simulink model "Drone_Sim"  (R2019b)
settings: Solver=ode15s  StartTime=0.0  StopTime=20  FixedStep=0.1
libraries: simulink x7
settings Model: Creator=harry  LastModifiedBy=cj
settings DataIOCC: ReturnWorkspaceOutputs=off
settings DebuggingCC: ArithmeticOperatorsInVariantConditions=warning
settings SFSimCC: CustomCodeUndefinedFunction=UseInterfaceOnly

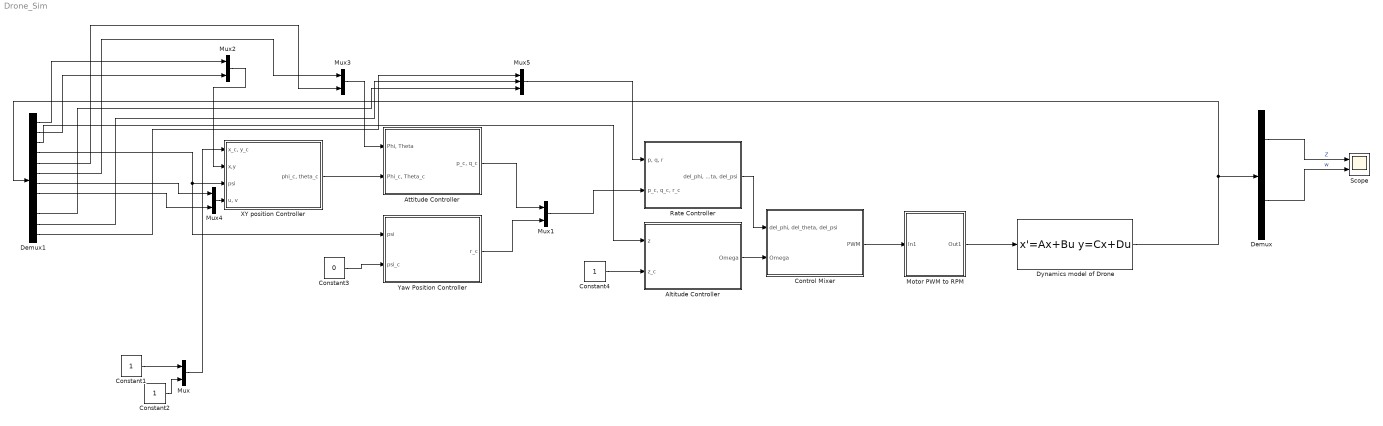
== system Drone_Sim ==
  Altitude Controller : Subsystem
  Attitude Controller : Subsystem
  Constant1 : Constant
  Constant2 : Constant
  Constant3 : Constant  Value=0
  Constant4 : Constant
  Control Mixer : Subsystem
  Demux : Demux  Outputs=12
  Demux1 : Demux  Outputs=12
  Dynamics model of Drone : StateSpace  A=[0,0,0,0,0,0,1,0,0,0,0,0;0,0,0,0,0,0,0,1,0,0,0,0;0,0,0,0,0,0,0,0,1,0,0,0;0,0,0,0,0,0,0,0,0,1,0,0;0,0,0,0,0,0,0,0,0,0,1,0;0,0,0,0,0,0,0,0,0,0,0,1;0,0,0,0,9.81000000000000,0,0,0,0,0,0,0;0,0,0,0,0,-9.81000000000000,0,0,0,0,0,0;0,0,0,0,0,0,0,0,0,0,0,0;0,0,0,0,0,0,0,0,0,0,0,0;0,0,0,0,0,0,0,0,0,0,0,0;0,0,0,0,0,0,0,0,0,0,0,0]  B=|  C=|  D=|  InitialCondition=[0,0,0,0,0,0,0,0,0,0,0,0]  ContinuousStateAttributes='X.Y.Z.Roll.PItch.Yaw.U.V.W.Roll_Rate.Pitch_Rate.Yaw_Rate'
      B=|
      | [ 0 0 0 0;
      |   0 0 0 0;
      |   0 0 0 0;
      |   0 0 0 0;
      |   0 0 0 0;
      |   0 0 0 0;
      |   0 0 0 0;
      |   0 0 0 0;    0.0002    0.0002    0.0002    0.0002;   -0.0731    0.0731   -0.0731    0.0731;   -0.1236    0.1236    0.1236   -0.1236;   -0.1272   -0.1272    0.1272    0.1272;]
      C=|
      | [1     0     0     0     0     0     0     0     0     0     0     0;
      |  0     1     0     0     0     0     0     0     0     0     0     0;
      |  0     0     1     0     0     0     0     0     0     0     0     0;
      |  0     0     0     1     0     0     0     0     0     0     0     0;
      |  0     0     0     0     1     0     0     0     0     0     0     0;
      |  0     0     0     0     0     1     0     0     0     0     0     0;
      |  0     0     0     0     0     0     1     0     0     0     0     0;
      |  0     0     0     0     0     0     0     1     0     0     0     0;
      |  0     0     0     0     0     0     0     0     1     0     0     0;
      |  0     0     0     0     0     0     0     0     0     1     0     0;
      |  0     0     0     0     0     0     0     0     0     0     1     0;
      |  0     0     0     0     0     0     0     0     0     0     0     1;]
      D=|
      | [0     0     0     0;
      |  0     0     0     0;
      |  0     0     0     0;
      |  0     0     0     0;
      |  0     0     0     0;
      |  0     0     0     0;
      |  0     0     0     0;
      |  0     0     0     0;
      |  0     0     0     0;
      |  0     0     0     0;
      |  0     0     0     0;
      |  0     0     0     0;]
  Motor PWM to RPM : Subsystem
  Mux{,1..4} (5 alike) : Mux  Inputs=2
  Mux5 : Mux  Inputs=3
  Rate Controller : Subsystem
  Scope : Scope  NumInputPorts=2
  XY position Controller : Subsystem
  "Yaw Position Controller " : Subsystem
  wires:
  Motor PWM to RPM/1(Out1) -> Dynamics model of Drone/1
  Control Mixer/1(PWM) -> Motor PWM to RPM/1(In1)
  Constant3/1 -> "Yaw Position Controller "/2(psi_c)
  Dynamics model of Drone/1 -> Demux1/1, Demux/1
  Demux/3 -> Scope/1  "Z"
  Demux/9 -> Scope/2  "w"
  Altitude Controller/1(Omega) -> Control Mixer/2(Omega)
  Rate Controller/1("del_phi, del_theta, del_psi") -> Control Mixer/1("del_phi, del_theta, del_psi")
  Attitude Controller/1("p_c, q_c") -> Mux1/1
  "Yaw Position Controller "/1(r_c) -> Mux1/2
  Mux1/1 -> Rate Controller/2("p_c, q_c, r_c")
  XY position Controller/1("phi_c, theta_c") -> Attitude Controller/2("Phi_c, Theta_c")
  Demux1/1 -> Mux2/1
  Mux2/1 -> XY position Controller/2(x,y)
  Demux1/2 -> Mux2/2
  Demux1/3 -> Altitude Controller/1(z)
  Demux1/4 -> XY position Controller/3(psi), "Yaw Position Controller "/1(psi)
  Demux1/5 -> Mux3/2
  Mux3/1 -> Attitude Controller/1("Phi, Theta")
  Demux1/6 -> Mux3/1
  Mux4/1 -> XY position Controller/4("u, v")
  Demux1/7 -> Mux4/1
  Demux1/8 -> Mux4/2
  Demux1/12 -> Mux5/1
  Demux1/11 -> Mux5/2
  Demux1/10 -> Mux5/3
  Mux5/1 -> Rate Controller/1("p, q, r")
  Mux/1 -> XY position Controller/1("x_c, y_c")
  Constant1/1 -> Mux/1
  Constant2/1 -> Mux/2
  Constant4/1 -> Altitude Controller/2(z_c)

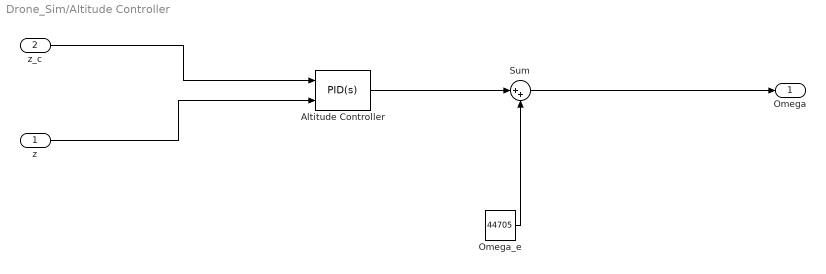
== system Drone_Sim/Altitude Controller ==
  z : Inport
  z_c : Inport  Port=2
  Altitude Controller : simulink/Continuous/PID Controller (2DOF)  Controller=PID  Form=Parallel  TimeDomain=Continuous-time  SampleTime=-1  IntegratorMethod=Forward Euler  FilterMethod=Forward Euler  ControllerParametersSource=internal  P=11000  I=3500  D=9000  UseFilter=on  N=100  b=1  c=1  TunerSelectOption=Transfer Function Based (PID Tuner App)  InitialConditionSource=internal  InitialConditionForIntegrator=0  InitialConditionForFilter=0  DifferentiatorICPrevScaledInput=0  ExternalReset=none  TrackingMode=off  Kt=1  LimitOutput=on  UpperSaturationLimit=15000  LowerSaturationLimit=-20000  LinearizeAsGain=on  AntiWindupMode=none  Kb=1  POutMin=[]  POutMax=[]  IOutMin=[]  IOutMax=[]  DOutMin=[]  DOutMax=[]  NOutMin=[]  NOutMax=[]  bOutMin=[]  bOutMax=[]  cOutMin=[]  cOutMax=[]  SumOutMin=[]  SumOutMax=[]  SaturationOutMin=[]  SaturationOutMax=[]  PParamMin=[]  PParamMax=[]  IParamMin=[]  IParamMax=[]  DParamMin=[]  DParamMax=[]  NParamMin=[]  NParamMax=[]  bParamMin=[]  bParamMax=[]  cParamMin=[]  cParamMax=[]  KbParamMin=[]  KbParamMax=[]  KtParamMin=[]  KtParamMax=[]  KbOutMin=[]  KbOutMax=[]  KtOutMin=[]  KtOutMax=[]  IntegratorOutMin=[]  IntegratorOutMax=[]  FilterOutMin=[]  FilterOutMax=[]  SumI1OutMin=[]  SumI1OutMax=[]  SumI2OutMin=[]  SumI2OutMax=[]  SumI3OutMin=[]  SumI3OutMax=[]  SumI4OutMin=[]  SumI4OutMax=[]  SumDOutMin=[]  SumDOutMax=[]  Sum1OutMin=[]  Sum1OutMax=[]  Sum2OutMin=[]  Sum2OutMax=[]  Sum3OutMin=[]  Sum3OutMax=[]  DifferentiatorOutMin=[]  DifferentiatorOutMax=[]  FilterDiffOutCoefMin=[]  FilterDiffOutCoefMax=[]  ReciprocalOutMin=[]  ReciprocalOutMax=[]  SumDenOutMin=[]  SumDenOutMax=[]  SumNumOutMin=[]  SumNumOutMax=[]  DivideOutMin=[]  DivideOutMax=[]  IntegratorContinuousStateAttributes=''  IntegratorStateMustResolveToSignalObject=off  IntegratorRTWStateStorageClass=Auto  FilterContinuousStateAttributes=''  FilterStateMustResolveToSignalObject=off  FilterRTWStateStorageClass=Auto  ParallelPVariant=InternalParameters  IdealPVariant=Disabled  IVariant=InternalParameters  DVariant=InternalParameters  bVariant=InternalParameters  cVariant=InternalParameters  IntegratorVariant=Continuous  SatVariant=Enabled  AWVariant=Passthrough  PCopyVariant=Disabled  TRVariant=Disabled  FdbkBlocksVariant=Forward  IdealPFdbkVariant=Disabled  SatFdbkVariant=Disabled  DerivativeFilterVariant=ContFilter  NVariant=InternalParameters  NCopyVariant=Disabled  FilterICVariant=InternalICsFilter  IntegratorICVariant=InternalICs  ExternalResetVariant=Disabled  TRSumVariant=Passthrough  SumFdbkVariant=Disabled  SumVariant=Sum_PID
  Omega_e : Constant  Value=44705
  Sum : Sum  Inputs=|++
  Omega : Outport  VectorParamsAs1DForOutWhenUnconnected=off
  wires:
  z/1 -> Altitude Controller/2
  z_c/1 -> Altitude Controller/1
  Sum/1 -> Omega/1
  Altitude Controller/1 -> Sum/1
  Omega_e/1 -> Sum/2

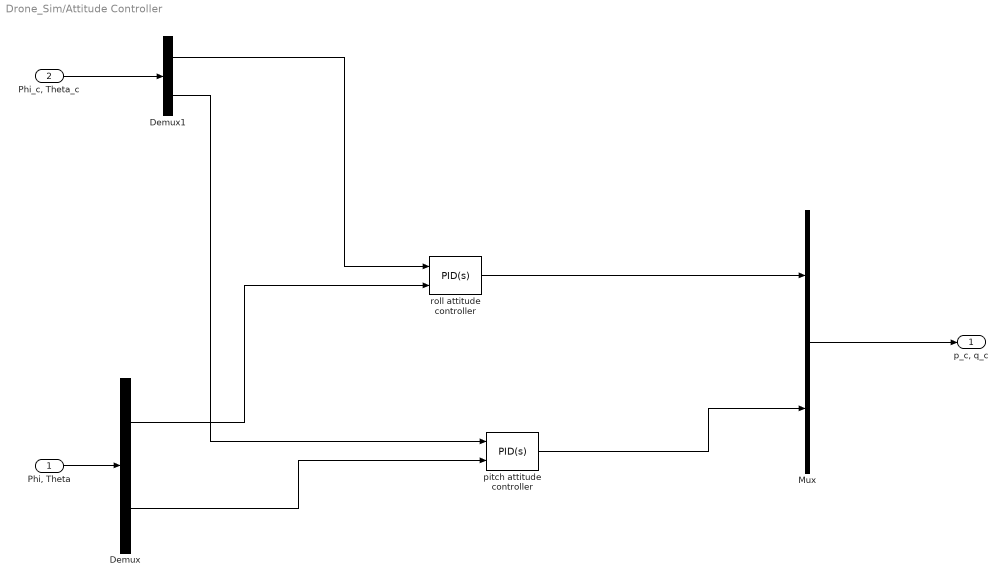
== system Drone_Sim/Attitude Controller ==
  "Phi, Theta" : Inport
  "Phi_c, Theta_c" : Inport  Port=2
  Demux : Demux  Outputs=2
  Demux1 : Demux  Outputs=2
  Mux : Mux  Inputs=2
  pitch attitude controller : simulink/Continuous/PID Controller (2DOF)  Controller=PID  Form=Parallel  TimeDomain=Continuous-time  SampleTime=-1  IntegratorMethod=Forward Euler  FilterMethod=Forward Euler  ControllerParametersSource=internal  P=3.5  I=2  D=0  UseFilter=on  N=100  b=1  c=1  TunerSelectOption=Transfer Function Based (PID Tuner App)  InitialConditionSource=internal  InitialConditionForIntegrator=0  InitialConditionForFilter=0  DifferentiatorICPrevScaledInput=0  ExternalReset=none  TrackingMode=off  Kt=1  LimitOutput=off  UpperSaturationLimit=inf  LowerSaturationLimit=-inf  LinearizeAsGain=on  AntiWindupMode=none  Kb=1  POutMin=[]  POutMax=[]  IOutMin=[]  IOutMax=[]  DOutMin=[]  DOutMax=[]  NOutMin=[]  NOutMax=[]  bOutMin=[]  bOutMax=[]  cOutMin=[]  cOutMax=[]  SumOutMin=[]  SumOutMax=[]  SaturationOutMin=[]  SaturationOutMax=[]  PParamMin=[]  PParamMax=[]  IParamMin=[]  IParamMax=[]  DParamMin=[]  DParamMax=[]  NParamMin=[]  NParamMax=[]  bParamMin=[]  bParamMax=[]  cParamMin=[]  cParamMax=[]  KbParamMin=[]  KbParamMax=[]  KtParamMin=[]  KtParamMax=[]  KbOutMin=[]  KbOutMax=[]  KtOutMin=[]  KtOutMax=[]  IntegratorOutMin=[]  IntegratorOutMax=[]  FilterOutMin=[]  FilterOutMax=[]  SumI1OutMin=[]  SumI1OutMax=[]  SumI2OutMin=[]  SumI2OutMax=[]  SumI3OutMin=[]  SumI3OutMax=[]  SumI4OutMin=[]  SumI4OutMax=[]  SumDOutMin=[]  SumDOutMax=[]  Sum1OutMin=[]  Sum1OutMax=[]  Sum2OutMin=[]  Sum2OutMax=[]  Sum3OutMin=[]  Sum3OutMax=[]  DifferentiatorOutMin=[]  DifferentiatorOutMax=[]  FilterDiffOutCoefMin=[]  FilterDiffOutCoefMax=[]  ReciprocalOutMin=[]  ReciprocalOutMax=[]  SumDenOutMin=[]  SumDenOutMax=[]  SumNumOutMin=[]  SumNumOutMax=[]  DivideOutMin=[]  DivideOutMax=[]  IntegratorContinuousStateAttributes=''  IntegratorStateMustResolveToSignalObject=off  IntegratorRTWStateStorageClass=Auto  FilterContinuousStateAttributes=''  FilterStateMustResolveToSignalObject=off  FilterRTWStateStorageClass=Auto  ParallelPVariant=InternalParameters  IdealPVariant=Disabled  IVariant=InternalParameters  DVariant=InternalParameters  bVariant=InternalParameters  cVariant=InternalParameters  IntegratorVariant=Continuous  SatVariant=Disabled  AWVariant=Passthrough  PCopyVariant=Disabled  TRVariant=Disabled  FdbkBlocksVariant=Forward  IdealPFdbkVariant=Disabled  SatFdbkVariant=Disabled  DerivativeFilterVariant=ContFilter  NVariant=InternalParameters  NCopyVariant=Disabled  FilterICVariant=InternalICsFilter  IntegratorICVariant=InternalICs  ExternalResetVariant=Disabled  TRSumVariant=Passthrough  SumFdbkVariant=Disabled  SumVariant=Sum_PID
  roll attitude controller : simulink/Continuous/PID Controller (2DOF)  Controller=PID  Form=Parallel  TimeDomain=Continuous-time  SampleTime=-1  IntegratorMethod=Forward Euler  FilterMethod=Forward Euler  ControllerParametersSource=internal  P=3.5  I=2  D=0  UseFilter=on  N=100  b=1  c=1  TunerSelectOption=Transfer Function Based (PID Tuner App)  InitialConditionSource=internal  InitialConditionForIntegrator=0  InitialConditionForFilter=0  DifferentiatorICPrevScaledInput=0  ExternalReset=none  TrackingMode=off  Kt=1  LimitOutput=off  UpperSaturationLimit=inf  LowerSaturationLimit=-inf  LinearizeAsGain=on  AntiWindupMode=none  Kb=1  POutMin=[]  POutMax=[]  IOutMin=[]  IOutMax=[]  DOutMin=[]  DOutMax=[]  NOutMin=[]  NOutMax=[]  bOutMin=[]  bOutMax=[]  cOutMin=[]  cOutMax=[]  SumOutMin=[]  SumOutMax=[]  SaturationOutMin=[]  SaturationOutMax=[]  PParamMin=[]  PParamMax=[]  IParamMin=[]  IParamMax=[]  DParamMin=[]  DParamMax=[]  NParamMin=[]  NParamMax=[]  bParamMin=[]  bParamMax=[]  cParamMin=[]  cParamMax=[]  KbParamMin=[]  KbParamMax=[]  KtParamMin=[]  KtParamMax=[]  KbOutMin=[]  KbOutMax=[]  KtOutMin=[]  KtOutMax=[]  IntegratorOutMin=[]  IntegratorOutMax=[]  FilterOutMin=[]  FilterOutMax=[]  SumI1OutMin=[]  SumI1OutMax=[]  SumI2OutMin=[]  SumI2OutMax=[]  SumI3OutMin=[]  SumI3OutMax=[]  SumI4OutMin=[]  SumI4OutMax=[]  SumDOutMin=[]  SumDOutMax=[]  Sum1OutMin=[]  Sum1OutMax=[]  Sum2OutMin=[]  Sum2OutMax=[]  Sum3OutMin=[]  Sum3OutMax=[]  DifferentiatorOutMin=[]  DifferentiatorOutMax=[]  FilterDiffOutCoefMin=[]  FilterDiffOutCoefMax=[]  ReciprocalOutMin=[]  ReciprocalOutMax=[]  SumDenOutMin=[]  SumDenOutMax=[]  SumNumOutMin=[]  SumNumOutMax=[]  DivideOutMin=[]  DivideOutMax=[]  IntegratorContinuousStateAttributes=''  IntegratorStateMustResolveToSignalObject=off  IntegratorRTWStateStorageClass=Auto  FilterContinuousStateAttributes=''  FilterStateMustResolveToSignalObject=off  FilterRTWStateStorageClass=Auto  ParallelPVariant=InternalParameters  IdealPVariant=Disabled  IVariant=InternalParameters  DVariant=InternalParameters  bVariant=InternalParameters  cVariant=InternalParameters  IntegratorVariant=Continuous  SatVariant=Disabled  AWVariant=Passthrough  PCopyVariant=Disabled  TRVariant=Disabled  FdbkBlocksVariant=Forward  IdealPFdbkVariant=Disabled  SatFdbkVariant=Disabled  DerivativeFilterVariant=ContFilter  NVariant=InternalParameters  NCopyVariant=Disabled  FilterICVariant=InternalICsFilter  IntegratorICVariant=InternalICs  ExternalResetVariant=Disabled  TRSumVariant=Passthrough  SumFdbkVariant=Disabled  SumVariant=Sum_PID
  "p_c, q_c" : Outport  VectorParamsAs1DForOutWhenUnconnected=off
  wires:
  "Phi, Theta"/1 -> Demux/1
  "Phi_c, Theta_c"/1 -> Demux1/1
  Mux/1 -> "p_c, q_c"/1
  Demux1/1 -> roll attitude controller/1
  Demux/1 -> roll attitude controller/2
  roll attitude controller/1 -> Mux/1
  Demux/2 -> pitch attitude controller/2
  Demux1/2 -> pitch attitude controller/1
  pitch attitude controller/1 -> Mux/2

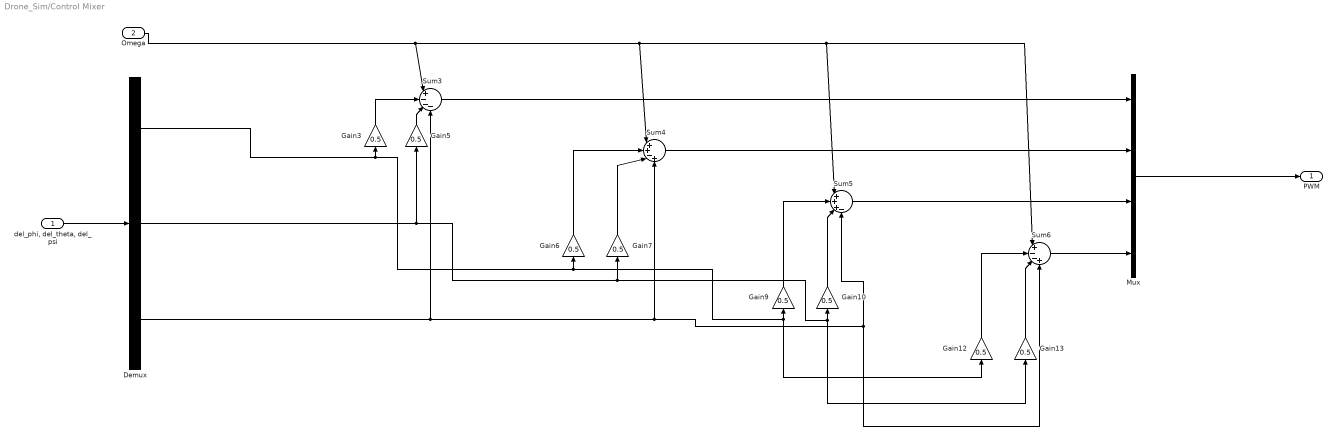
== system Drone_Sim/Control Mixer ==
  "del_phi, del_theta, del_psi" : Inport
  Omega : Inport  Port=2
  Demux : Demux  Outputs=3
  Gain{3,5..7,9..10,12..13} (8 alike) : Gain  Gain=0.5
  Mux : Mux
  Sum3 : Sum  Inputs=|+---
  Sum4 : Sum  Inputs=|++-+
  Sum5 : Sum  Inputs=|+++-
  Sum6 : Sum  Inputs=|+--+
  PWM : Outport  VectorParamsAs1DForOutWhenUnconnected=off
  wires:
  "del_phi, del_theta, del_psi"/1 -> Demux/1
  Omega/1 -> Sum6/1, Sum5/1, Sum4/1, Sum3/1
  Gain3/1 -> Sum3/2
  Sum3/1 -> Mux/1
  Gain7/1 -> Sum4/3
  Gain6/1 -> Sum4/2
  Gain10/1 -> Sum5/3
  Gain9/1 -> Sum5/2
  Sum4/1 -> Mux/2
  Sum5/1 -> Mux/3
  Gain13/1 -> Sum6/3
  Gain12/1 -> Sum6/2
  Demux/3 -> Sum3/4, Sum5/4, Sum6/4, Sum4/4
  Sum6/1 -> Mux/4
  Mux/1 -> PWM/1
  Demux/1 -> Gain9/1, Gain12/1, Gain6/1, Gain3/1
  Demux/2 -> Gain10/1, Gain13/1, Gain7/1, Gain5/1
  Gain5/1 -> Sum3/3

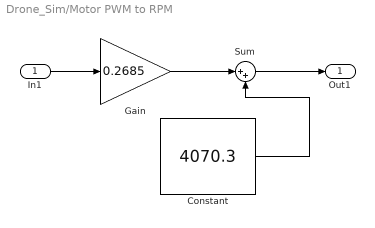
== system Drone_Sim/Motor PWM to RPM ==
  In1 : Inport
  Constant : Constant  Value=4070.3
  Gain : Gain  Gain=0.2685
  Sum : Sum  Inputs=|++
  Out1 : Outport  VectorParamsAs1DForOutWhenUnconnected=off
  wires:
  In1/1 -> Gain/1
  Gain/1 -> Sum/1
  Constant/1 -> Sum/2
  Sum/1 -> Out1/1

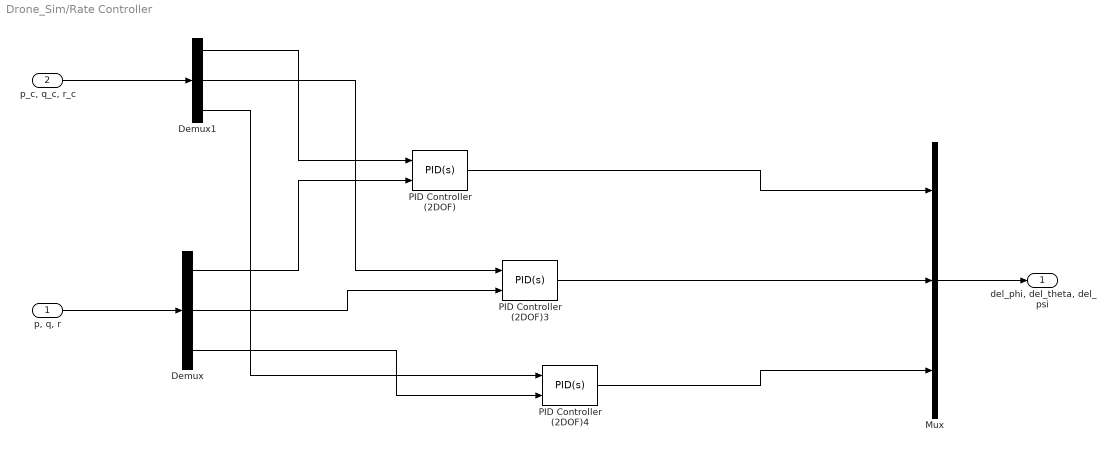
== system Drone_Sim/Rate Controller ==
  "p, q, r" : Inport
  "p_c, q_c, r_c" : Inport  Port=2
  Demux : Demux  Outputs=3
  Demux1 : Demux  Outputs=3
  Mux : Mux  Inputs=3
  PID Controller (2DOF) : simulink/Continuous/PID Controller (2DOF)  Controller=PID  Form=Parallel  TimeDomain=Continuous-time  SampleTime=-1  IntegratorMethod=Forward Euler  FilterMethod=Forward Euler  ControllerParametersSource=internal  P=70  I=0  D=0  UseFilter=on  N=100  b=1  c=1  TunerSelectOption=Transfer Function Based (PID Tuner App)  InitialConditionSource=internal  InitialConditionForIntegrator=0  InitialConditionForFilter=0  DifferentiatorICPrevScaledInput=0  ExternalReset=none  TrackingMode=off  Kt=1  LimitOutput=off  UpperSaturationLimit=inf  LowerSaturationLimit=-inf  LinearizeAsGain=on  AntiWindupMode=none  Kb=1  POutMin=[]  POutMax=[]  IOutMin=[]  IOutMax=[]  DOutMin=[]  DOutMax=[]  NOutMin=[]  NOutMax=[]  bOutMin=[]  bOutMax=[]  cOutMin=[]  cOutMax=[]  SumOutMin=[]  SumOutMax=[]  SaturationOutMin=[]  SaturationOutMax=[]  PParamMin=[]  PParamMax=[]  IParamMin=[]  IParamMax=[]  DParamMin=[]  DParamMax=[]  NParamMin=[]  NParamMax=[]  bParamMin=[]  bParamMax=[]  cParamMin=[]  cParamMax=[]  KbParamMin=[]  KbParamMax=[]  KtParamMin=[]  KtParamMax=[]  KbOutMin=[]  KbOutMax=[]  KtOutMin=[]  KtOutMax=[]  IntegratorOutMin=[]  IntegratorOutMax=[]  FilterOutMin=[]  FilterOutMax=[]  SumI1OutMin=[]  SumI1OutMax=[]  SumI2OutMin=[]  SumI2OutMax=[]  SumI3OutMin=[]  SumI3OutMax=[]  SumI4OutMin=[]  SumI4OutMax=[]  SumDOutMin=[]  SumDOutMax=[]  Sum1OutMin=[]  Sum1OutMax=[]  Sum2OutMin=[]  Sum2OutMax=[]  Sum3OutMin=[]  Sum3OutMax=[]  DifferentiatorOutMin=[]  DifferentiatorOutMax=[]  FilterDiffOutCoefMin=[]  FilterDiffOutCoefMax=[]  ReciprocalOutMin=[]  ReciprocalOutMax=[]  SumDenOutMin=[]  SumDenOutMax=[]  SumNumOutMin=[]  SumNumOutMax=[]  DivideOutMin=[]  DivideOutMax=[]  IntegratorContinuousStateAttributes=''  IntegratorStateMustResolveToSignalObject=off  IntegratorRTWStateStorageClass=Auto  FilterContinuousStateAttributes=''  FilterStateMustResolveToSignalObject=off  FilterRTWStateStorageClass=Auto  ParallelPVariant=InternalParameters  IdealPVariant=Disabled  IVariant=InternalParameters  DVariant=InternalParameters  bVariant=InternalParameters  cVariant=InternalParameters  IntegratorVariant=Continuous  SatVariant=Disabled  AWVariant=Passthrough  PCopyVariant=Disabled  TRVariant=Disabled  FdbkBlocksVariant=Forward  IdealPFdbkVariant=Disabled  SatFdbkVariant=Disabled  DerivativeFilterVariant=ContFilter  NVariant=InternalParameters  NCopyVariant=Disabled  FilterICVariant=InternalICsFilter  IntegratorICVariant=InternalICs  ExternalResetVariant=Disabled  TRSumVariant=Passthrough  SumFdbkVariant=Disabled  SumVariant=Sum_PID
  PID Controller (2DOF)3 : simulink/Continuous/PID Controller (2DOF)  Controller=PID  Form=Parallel  TimeDomain=Continuous-time  SampleTime=-1  IntegratorMethod=Forward Euler  FilterMethod=Forward Euler  ControllerParametersSource=internal  P=70  I=0  D=0  UseFilter=on  N=100  b=1  c=1  TunerSelectOption=Transfer Function Based (PID Tuner App)  InitialConditionSource=internal  InitialConditionForIntegrator=0  InitialConditionForFilter=0  DifferentiatorICPrevScaledInput=0  ExternalReset=none  TrackingMode=off  Kt=1  LimitOutput=off  UpperSaturationLimit=inf  LowerSaturationLimit=-inf  LinearizeAsGain=on  AntiWindupMode=none  Kb=1  POutMin=[]  POutMax=[]  IOutMin=[]  IOutMax=[]  DOutMin=[]  DOutMax=[]  NOutMin=[]  NOutMax=[]  bOutMin=[]  bOutMax=[]  cOutMin=[]  cOutMax=[]  SumOutMin=[]  SumOutMax=[]  SaturationOutMin=[]  SaturationOutMax=[]  PParamMin=[]  PParamMax=[]  IParamMin=[]  IParamMax=[]  DParamMin=[]  DParamMax=[]  NParamMin=[]  NParamMax=[]  bParamMin=[]  bParamMax=[]  cParamMin=[]  cParamMax=[]  KbParamMin=[]  KbParamMax=[]  KtParamMin=[]  KtParamMax=[]  KbOutMin=[]  KbOutMax=[]  KtOutMin=[]  KtOutMax=[]  IntegratorOutMin=[]  IntegratorOutMax=[]  FilterOutMin=[]  FilterOutMax=[]  SumI1OutMin=[]  SumI1OutMax=[]  SumI2OutMin=[]  SumI2OutMax=[]  SumI3OutMin=[]  SumI3OutMax=[]  SumI4OutMin=[]  SumI4OutMax=[]  SumDOutMin=[]  SumDOutMax=[]  Sum1OutMin=[]  Sum1OutMax=[]  Sum2OutMin=[]  Sum2OutMax=[]  Sum3OutMin=[]  Sum3OutMax=[]  DifferentiatorOutMin=[]  DifferentiatorOutMax=[]  FilterDiffOutCoefMin=[]  FilterDiffOutCoefMax=[]  ReciprocalOutMin=[]  ReciprocalOutMax=[]  SumDenOutMin=[]  SumDenOutMax=[]  SumNumOutMin=[]  SumNumOutMax=[]  DivideOutMin=[]  DivideOutMax=[]  IntegratorContinuousStateAttributes=''  IntegratorStateMustResolveToSignalObject=off  IntegratorRTWStateStorageClass=Auto  FilterContinuousStateAttributes=''  FilterStateMustResolveToSignalObject=off  FilterRTWStateStorageClass=Auto  ParallelPVariant=InternalParameters  IdealPVariant=Disabled  IVariant=InternalParameters  DVariant=InternalParameters  bVariant=InternalParameters  cVariant=InternalParameters  IntegratorVariant=Continuous  SatVariant=Disabled  AWVariant=Passthrough  PCopyVariant=Disabled  TRVariant=Disabled  FdbkBlocksVariant=Forward  IdealPFdbkVariant=Disabled  SatFdbkVariant=Disabled  DerivativeFilterVariant=ContFilter  NVariant=InternalParameters  NCopyVariant=Disabled  FilterICVariant=InternalICsFilter  IntegratorICVariant=InternalICs  ExternalResetVariant=Disabled  TRSumVariant=Passthrough  SumFdbkVariant=Disabled  SumVariant=Sum_PID
  PID Controller (2DOF)4 : simulink/Continuous/PID Controller (2DOF)  Controller=PID  Form=Parallel  TimeDomain=Continuous-time  SampleTime=-1  IntegratorMethod=Forward Euler  FilterMethod=Forward Euler  ControllerParametersSource=internal  P=70  I=16.70  D=0  UseFilter=on  N=100  b=1  c=1  TunerSelectOption=Transfer Function Based (PID Tuner App)  InitialConditionSource=internal  InitialConditionForIntegrator=0  InitialConditionForFilter=0  DifferentiatorICPrevScaledInput=0  ExternalReset=none  TrackingMode=off  Kt=1  LimitOutput=off  UpperSaturationLimit=inf  LowerSaturationLimit=-inf  LinearizeAsGain=on  AntiWindupMode=none  Kb=1  POutMin=[]  POutMax=[]  IOutMin=[]  IOutMax=[]  DOutMin=[]  DOutMax=[]  NOutMin=[]  NOutMax=[]  bOutMin=[]  bOutMax=[]  cOutMin=[]  cOutMax=[]  SumOutMin=[]  SumOutMax=[]  SaturationOutMin=[]  SaturationOutMax=[]  PParamMin=[]  PParamMax=[]  IParamMin=[]  IParamMax=[]  DParamMin=[]  DParamMax=[]  NParamMin=[]  NParamMax=[]  bParamMin=[]  bParamMax=[]  cParamMin=[]  cParamMax=[]  KbParamMin=[]  KbParamMax=[]  KtParamMin=[]  KtParamMax=[]  KbOutMin=[]  KbOutMax=[]  KtOutMin=[]  KtOutMax=[]  IntegratorOutMin=[]  IntegratorOutMax=[]  FilterOutMin=[]  FilterOutMax=[]  SumI1OutMin=[]  SumI1OutMax=[]  SumI2OutMin=[]  SumI2OutMax=[]  SumI3OutMin=[]  SumI3OutMax=[]  SumI4OutMin=[]  SumI4OutMax=[]  SumDOutMin=[]  SumDOutMax=[]  Sum1OutMin=[]  Sum1OutMax=[]  Sum2OutMin=[]  Sum2OutMax=[]  Sum3OutMin=[]  Sum3OutMax=[]  DifferentiatorOutMin=[]  DifferentiatorOutMax=[]  FilterDiffOutCoefMin=[]  FilterDiffOutCoefMax=[]  ReciprocalOutMin=[]  ReciprocalOutMax=[]  SumDenOutMin=[]  SumDenOutMax=[]  SumNumOutMin=[]  SumNumOutMax=[]  DivideOutMin=[]  DivideOutMax=[]  IntegratorContinuousStateAttributes=''  IntegratorStateMustResolveToSignalObject=off  IntegratorRTWStateStorageClass=Auto  FilterContinuousStateAttributes=''  FilterStateMustResolveToSignalObject=off  FilterRTWStateStorageClass=Auto  ParallelPVariant=InternalParameters  IdealPVariant=Disabled  IVariant=InternalParameters  DVariant=InternalParameters  bVariant=InternalParameters  cVariant=InternalParameters  IntegratorVariant=Continuous  SatVariant=Disabled  AWVariant=Passthrough  PCopyVariant=Disabled  TRVariant=Disabled  FdbkBlocksVariant=Forward  IdealPFdbkVariant=Disabled  SatFdbkVariant=Disabled  DerivativeFilterVariant=ContFilter  NVariant=InternalParameters  NCopyVariant=Disabled  FilterICVariant=InternalICsFilter  IntegratorICVariant=InternalICs  ExternalResetVariant=Disabled  TRSumVariant=Passthrough  SumFdbkVariant=Disabled  SumVariant=Sum_PID
  "del_phi, del_theta, del_psi" : Outport  VectorParamsAs1DForOutWhenUnconnected=off
  wires:
  "p, q, r"/1 -> Demux/1
  "p_c, q_c, r_c"/1 -> Demux1/1
  Mux/1 -> "del_phi, del_theta, del_psi"/1
  Demux1/1 -> PID Controller (2DOF)/1
  Demux/1 -> PID Controller (2DOF)/2
  Demux1/2 -> PID Controller (2DOF)3/1
  Demux/2 -> PID Controller (2DOF)3/2
  Demux1/3 -> PID Controller (2DOF)4/1
  Demux/3 -> PID Controller (2DOF)4/2
  PID Controller (2DOF)/1 -> Mux/1
  PID Controller (2DOF)3/1 -> Mux/2
  PID Controller (2DOF)4/1 -> Mux/3

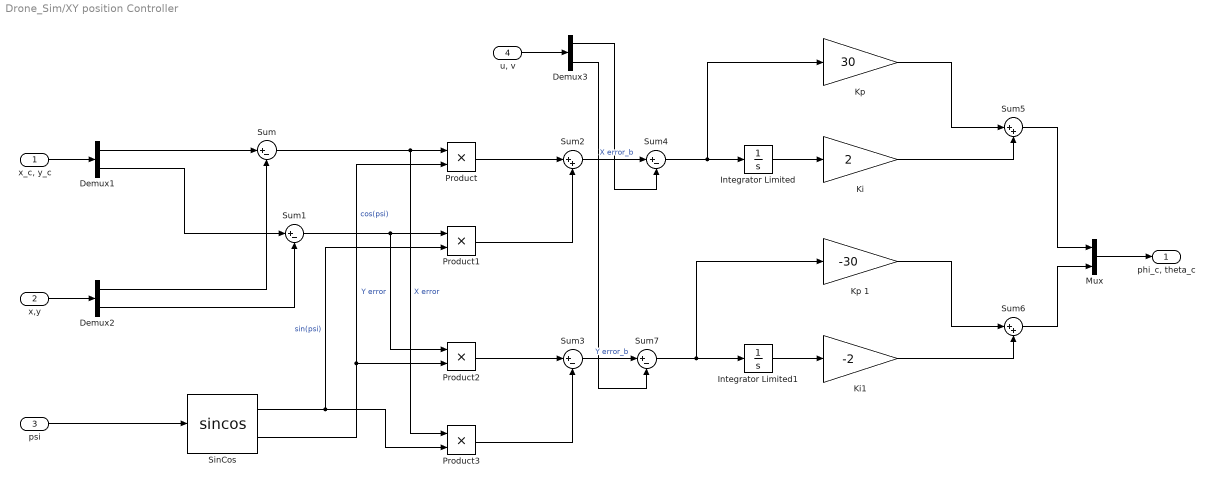
== system Drone_Sim/XY position Controller ==
  "x_c, y_c" : Inport
  x,y : Inport  Port=2
  psi : Inport  Port=3
  "u, v" : Inport  Port=4
  Demux1 : Demux  Outputs=2
  Demux2 : Demux  Outputs=2
  Demux3 : Demux  Outputs=2
  Integrator Limited : Integrator  LimitOutput=on  UpperSaturationLimit=30  LowerSaturationLimit=-30
  Integrator Limited1 : Integrator  LimitOutput=on  UpperSaturationLimit=30  LowerSaturationLimit=-30
  Ki : Gain  Gain=2
  Ki1 : Gain  Gain=-2
  "Kp " : Gain  Gain=30
  Kp 1 : Gain  Gain=-30
  Mux : Mux  Inputs=2
  Product{,1..3} (4 alike) : Product
  SinCos : Trigonometry  Operator=sincos
  Sum{,1,3..4,7} (5 alike) : Sum  Inputs=|+-
  Sum2 : Sum  Inputs=|++
  Sum5 : Sum  Inputs=|++
  Sum6 : Sum  Inputs=|++
  "phi_c, theta_c" : Outport  VectorParamsAs1DForOutWhenUnconnected=off
  wires:
  "x_c, y_c"/1 -> Demux1/1
  x,y/1 -> Demux2/1
  "u, v"/1 -> Demux3/1
  Demux1/1 -> Sum/1
  Demux2/1 -> Sum/2
  Sum/1 -> Product3/1, Product/1  "X error"
  psi/1 -> SinCos/1
  SinCos/2 -> Product2/2, Product/2  "cos(psi)"
  Demux1/2 -> Sum1/1
  Demux2/2 -> Sum1/2
  Sum1/1 -> Product2/1, Product1/1  "Y error"
  SinCos/1 -> Product1/2, Product3/2  "sin(psi)"
  Product/1 -> Sum2/1
  Product1/1 -> Sum2/2
  Product2/1 -> Sum3/1
  Product3/1 -> Sum3/2
  Sum2/1 -> Sum4/1  "X error_b"
  Demux3/1 -> Sum4/2
  Sum4/1 -> "Kp "/1, Integrator Limited/1
  Integrator Limited/1 -> Ki/1
  Integrator Limited1/1 -> Ki1/1
  "Kp "/1 -> Sum5/1
  Ki/1 -> Sum5/2
  Sum5/1 -> Mux/1
  Ki1/1 -> Sum6/2
  Kp 1/1 -> Sum6/1
  Sum6/1 -> Mux/2
  Mux/1 -> "phi_c, theta_c"/1
  Sum3/1 -> Sum7/1  "Y error_b"
  Demux3/2 -> Sum7/2
  Sum7/1 -> Kp 1/1, Integrator Limited1/1

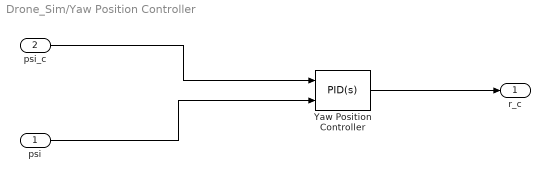
== system Drone_Sim/Yaw Position Controller  ==
  psi : Inport
  psi_c : Inport  Port=2
  Yaw Position Controller : simulink/Continuous/PID Controller (2DOF)  Controller=PID  Form=Parallel  TimeDomain=Continuous-time  SampleTime=-1  IntegratorMethod=Forward Euler  FilterMethod=Forward Euler  ControllerParametersSource=internal  P=3  I=0  D=0  UseFilter=on  N=100  b=1  c=1  TunerSelectOption=Transfer Function Based (PID Tuner App)  InitialConditionSource=internal  InitialConditionForIntegrator=0  InitialConditionForFilter=0  DifferentiatorICPrevScaledInput=0  ExternalReset=none  TrackingMode=off  Kt=1  LimitOutput=on  UpperSaturationLimit=200  LowerSaturationLimit=-200  LinearizeAsGain=on  AntiWindupMode=none  Kb=1  POutMin=[]  POutMax=[]  IOutMin=[]  IOutMax=[]  DOutMin=[]  DOutMax=[]  NOutMin=[]  NOutMax=[]  bOutMin=[]  bOutMax=[]  cOutMin=[]  cOutMax=[]  SumOutMin=[]  SumOutMax=[]  SaturationOutMin=[]  SaturationOutMax=[]  PParamMin=[]  PParamMax=[]  IParamMin=[]  IParamMax=[]  DParamMin=[]  DParamMax=[]  NParamMin=[]  NParamMax=[]  bParamMin=[]  bParamMax=[]  cParamMin=[]  cParamMax=[]  KbParamMin=[]  KbParamMax=[]  KtParamMin=[]  KtParamMax=[]  KbOutMin=[]  KbOutMax=[]  KtOutMin=[]  KtOutMax=[]  IntegratorOutMin=[]  IntegratorOutMax=[]  FilterOutMin=[]  FilterOutMax=[]  SumI1OutMin=[]  SumI1OutMax=[]  SumI2OutMin=[]  SumI2OutMax=[]  SumI3OutMin=[]  SumI3OutMax=[]  SumI4OutMin=[]  SumI4OutMax=[]  SumDOutMin=[]  SumDOutMax=[]  Sum1OutMin=[]  Sum1OutMax=[]  Sum2OutMin=[]  Sum2OutMax=[]  Sum3OutMin=[]  Sum3OutMax=[]  DifferentiatorOutMin=[]  DifferentiatorOutMax=[]  FilterDiffOutCoefMin=[]  FilterDiffOutCoefMax=[]  ReciprocalOutMin=[]  ReciprocalOutMax=[]  SumDenOutMin=[]  SumDenOutMax=[]  SumNumOutMin=[]  SumNumOutMax=[]  DivideOutMin=[]  DivideOutMax=[]  IntegratorContinuousStateAttributes=''  IntegratorStateMustResolveToSignalObject=off  IntegratorRTWStateStorageClass=Auto  FilterContinuousStateAttributes=''  FilterStateMustResolveToSignalObject=off  FilterRTWStateStorageClass=Auto  ParallelPVariant=InternalParameters  IdealPVariant=Disabled  IVariant=InternalParameters  DVariant=InternalParameters  bVariant=InternalParameters  cVariant=InternalParameters  IntegratorVariant=Continuous  SatVariant=Enabled  AWVariant=Passthrough  PCopyVariant=Disabled  TRVariant=Disabled  FdbkBlocksVariant=Forward  IdealPFdbkVariant=Disabled  SatFdbkVariant=Disabled  DerivativeFilterVariant=ContFilter  NVariant=InternalParameters  NCopyVariant=Disabled  FilterICVariant=InternalICsFilter  IntegratorICVariant=InternalICs  ExternalResetVariant=Disabled  TRSumVariant=Passthrough  SumFdbkVariant=Disabled  SumVariant=Sum_PID
  r_c : Outport  VectorParamsAs1DForOutWhenUnconnected=off
  wires:
  psi/1 -> Yaw Position Controller/2
  psi_c/1 -> Yaw Position Controller/1
  Yaw Position Controller/1 -> r_c/1
